simulink model "Tut17_TriggeredSubsystem_Part2"  (R2021a)
settings: Solver=FixedStepDiscrete  StartTime=0.0  StopTime=30  FixedStep=1  RelTol=1e-3
libraries: simulink x1
settings Model: Creator=cheta  LastModifiedBy=cheta

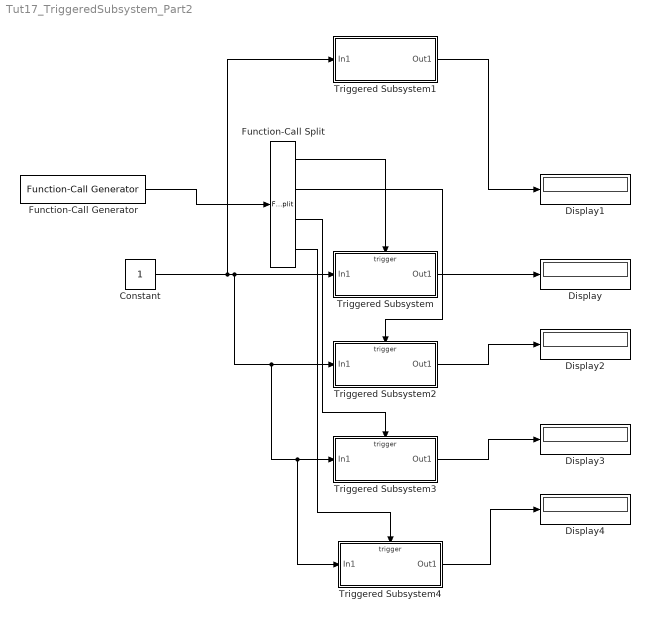
== system Tut17_TriggeredSubsystem_Part2 ==
  Constant : Constant
  Display{,1..4} (5 alike) : Display
  Function-Call Generator : simulink/Ports & Subsystems/Function-Call Generator  sample_time=3  numberOfIterations=1  DisallowWideOutput=off
  Function-Call Split : FunctionCallSplit  IconShape=distinctive  NumOutputPorts=4  OutputPortLayout=default
  Triggered Subsystem : Subsystem  TreatAsAtomicUnit=on
  Triggered Subsystem1 : Subsystem  TreatAsAtomicUnit=on  SystemSampleTime=1
  Triggered Subsystem2 : Subsystem  TreatAsAtomicUnit=on
  Triggered Subsystem3 : Subsystem  TreatAsAtomicUnit=on
  Triggered Subsystem4 : Subsystem  TreatAsAtomicUnit=on
  wires:
  Constant/1 -> Triggered Subsystem1/1(In1), Triggered Subsystem4/1(In1), Triggered Subsystem3/1(In1), Triggered Subsystem2/1(In1), Triggered Subsystem/1(In1)
  Triggered Subsystem/1(Out1) -> Display/1
  Function-Call Generator/1 -> Function-Call Split/1
  Triggered Subsystem1/1(Out1) -> Display1/1
  Triggered Subsystem2/1(Out1) -> Display2/1
  Triggered Subsystem3/1(Out1) -> Display3/1
  Triggered Subsystem4/1(Out1) -> Display4/1
  Function-Call Split/1 -> Triggered Subsystem/Trigger
  Function-Call Split/2 -> Triggered Subsystem2/Trigger
  Function-Call Split/3 -> Triggered Subsystem3/Trigger
  Function-Call Split/4 -> Triggered Subsystem4/Trigger

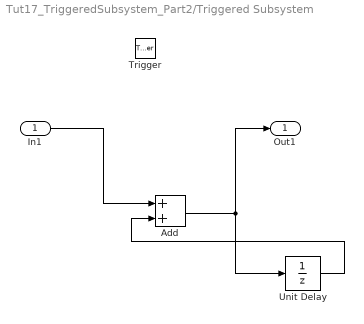
== system Tut17_TriggeredSubsystem_Part2/Triggered Subsystem ==
  In1 : Inport
  Trigger : TriggerPort  TriggerType=function-call  VariantControl=(inherit)
  Add : Sum
  Unit Delay : UnitDelay  SampleTime=-1  HasFrameUpgradeWarning=on
  Out1 : Outport
  wires:
  In1/1 -> Add/1
  Unit Delay/1 -> Add/2
  Add/1 -> Unit Delay/1, Out1/1

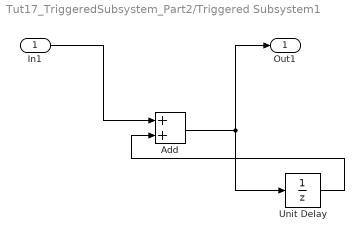
== system Tut17_TriggeredSubsystem_Part2/Triggered Subsystem1 ==
  In1 : Inport
  Add : Sum
  Unit Delay : UnitDelay  SampleTime=-1  HasFrameUpgradeWarning=on
  Out1 : Outport
  wires:
  Add/1 -> Out1/1, Unit Delay/1
  Unit Delay/1 -> Add/2
  In1/1 -> Add/1

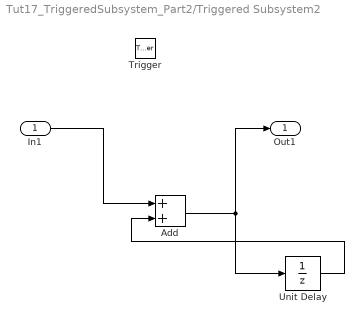
== system Tut17_TriggeredSubsystem_Part2/Triggered Subsystem2 ==
  In1 : Inport
  Trigger : TriggerPort  TriggerType=function-call  VariantControl=(inherit)
  Add : Sum
  Unit Delay : UnitDelay  SampleTime=-1  HasFrameUpgradeWarning=on
  Out1 : Outport
  wires:
  Add/1 -> Out1/1, Unit Delay/1
  Unit Delay/1 -> Add/2
  In1/1 -> Add/1

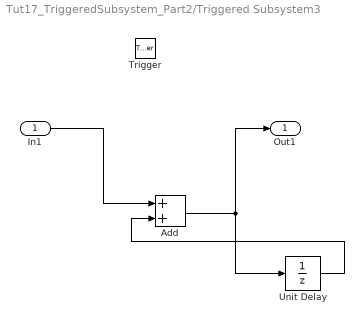
== system Tut17_TriggeredSubsystem_Part2/Triggered Subsystem3 ==
  In1 : Inport
  Trigger : TriggerPort  TriggerType=function-call  VariantControl=(inherit)
  Add : Sum
  Unit Delay : UnitDelay  SampleTime=-1  HasFrameUpgradeWarning=on
  Out1 : Outport
  wires:
  In1/1 -> Add/1
  Unit Delay/1 -> Add/2
  Add/1 -> Unit Delay/1, Out1/1

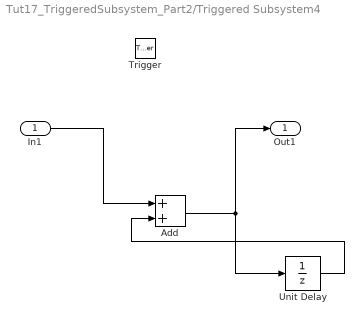
== system Tut17_TriggeredSubsystem_Part2/Triggered Subsystem4 ==
  In1 : Inport
  Trigger : TriggerPort  TriggerType=function-call  VariantControl=(inherit)
  Add : Sum
  Unit Delay : UnitDelay  SampleTime=-1  HasFrameUpgradeWarning=on
  Out1 : Outport
  wires:
  Add/1 -> Out1/1, Unit Delay/1
  Unit Delay/1 -> Add/2
  In1/1 -> Add/1
